simulink subsystem "environmentModel"  (R2026a)
settings: Solver=VariableStepAuto
values from neighbouring files (symbols this model uses):
  envParams : value not decoded    [plantParams.sldd]
  vehicleParams = 18.0    [plantParams.sldd]
libraries: simulink x1, aerolibatmos2 x1, aerolibutil x1
settings Model: DataDictionary=plantParams.sldd  EnableAccessToBaseWorkspace=off  Creator=maxhu  LastModifiedBy=maxhu

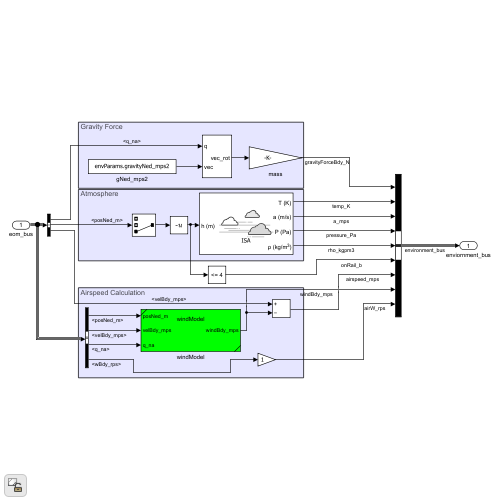
[thumbnail: Simulink's stored preview of the top-level diagram]
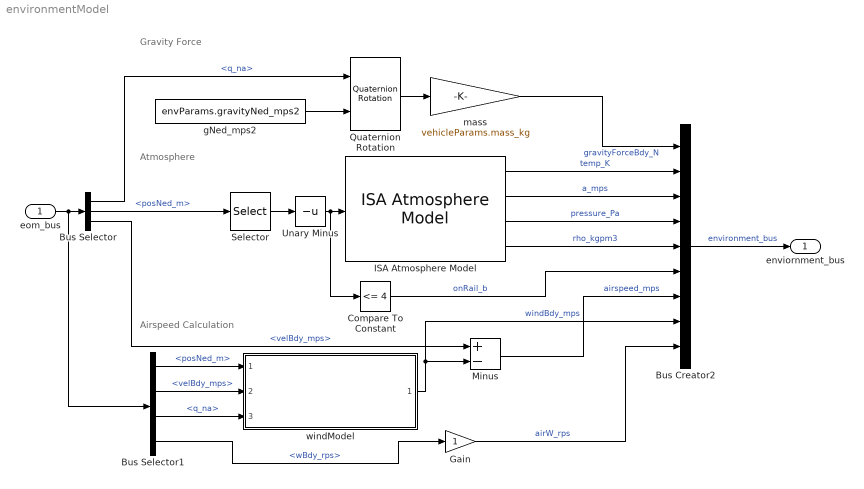
== system environmentModel ==
  note: Atmosphere
  note: Gravity Force
  note: Airspeed Calculation
  eom_bus : Inport
  Bus Creator2 : BusCreator  Inputs=9
  Bus Selector : BusSelector  OutputSignals=q_na,posNed_m,velBdy_mps
  Bus Selector1 : BusSelector  OutputSignals=posNed_m,velBdy_mps,q_na,wBdy_rps
  Compare To Constant : simulink/Logic and Bit Operations/Compare To Constant  relop=<=  const=4  OutDataTypeStr=boolean
  Gain : Gain
  ISA Atmosphere Model : aerolibatmos2/ISA Atmosphere Model  useExtended=off  action=None  custom=off  viscosityOut=off  g=9.80665  gamma=1.4  R=287.0531  L=0.0065  h_trop=11000  h_strat=20000  rho0=1.225  P0=101325  T0=288.15  h0=0  S=110.4  Tref=273.15  muref=1.716e-5
  Minus : Sum  Inputs=+-
  Quaternion Rotation : aerolibutil/Quaternion Rotation
  Selector : Selector  InputPortWidth=3  IndexOptions=Index vector (dialog)  Indices=[3]  OutputSizes=1
  Unary Minus : UnaryMinus
  gNed_mps2 : Constant  Value=envParams.gravityNed_mps2
  mass : Gain  Gain=vehicleParams.mass_kg
  windModel : Subsystem  ReferencedSubsystem=windModel
      settings: PermitHierarchicalResolution=None
  enviornment_bus : Outport
  wires:
  Bus Selector1/4 -> Gain/1  "<wBdy_rps>"
  Gain/1 -> Bus Creator2/9  "airW_rps"
  Bus Selector1/3 -> windModel/3  "<q_na>"
  windModel/1 -> Minus/2, Bus Creator2/8  "windBdy_mps"
  Bus Selector1/1 -> windModel/1  "<posNed_m>"
  Bus Selector1/2 -> windModel/2  "<velBdy_mps>"
  Minus/1 -> Bus Creator2/7  "airspeed_mps"
  Bus Selector/3 -> Minus/1  "<velBdy_mps>"
  eom_bus/1 -> Bus Selector1/1, Bus Selector/1
  Bus Creator2/1 -> enviornment_bus/1  "environment_bus"
  Bus Selector/1 -> Quaternion Rotation/1  "<q_na>"
  ISA Atmosphere Model/3 -> Bus Creator2/4  "pressure_Pa"
  ISA Atmosphere Model/1 -> Bus Creator2/2  "temp_K"
  Selector/1 -> Unary Minus/1
  Bus Selector/2 -> Selector/1  "<posNed_m>"
  Quaternion Rotation/1 -> mass/1
  ISA Atmosphere Model/4 -> Bus Creator2/5  "rho_kgpm3"
  gNed_mps2/1 -> Quaternion Rotation/2
  Unary Minus/1 -> ISA Atmosphere Model/1, Compare To Constant/1
  mass/1 -> Bus Creator2/1  "gravityForceBdy_N"
  ISA Atmosphere Model/2 -> Bus Creator2/3  "a_mps"
  Compare To Constant/1 -> Bus Creator2/6  "onRail_b"
